simulink model "pfb_fir_generic_test_sim3"  (R2012b)
settings: Solver=VariableStepDiscrete  StartTime=0.0  StopTime=10.0  RelTol=1e-3
model workspace (MAT data in the model file):
  synci = [0 1 2 3 4 5 6 7 8 9 10 11 ... (589826 elements, 294913x2)]
  din0 = [0 1 2 3 4 5 6 7 8 9 10 11 ... (73730 elements, 36865x2)]
  din1 = [0 1 2 3 4 5 6 7 8 9 10 11 ... (73730 elements, 36865x2)]
  din2 = [0 1 2 3 4 5 6 7 8 9 10 11 ... (73730 elements, 36865x2)]
  din3 = [0 1 2 3 4 5 6 7 8 9 10 11 ... (73730 elements, 36865x2)]
  din4 = [0 1 2 3 4 5 6 7 8 9 10 11 ... (73730 elements, 36865x2)]
  din5 = [0 1 2 3 4 5 6 7 8 9 10 11 ... (73730 elements, 36865x2)]
  din6 = [0 1 2 3 4 5 6 7 8 9 10 11 ... (73730 elements, 36865x2)]
  din7 = [0 1 2 3 4 5 6 7 8 9 10 11 ... (73730 elements, 36865x2)]
libraries: xbsIndex_r4 x5585, casper_library_delays x1
(part 13 of 25)

== system pfb_fir_generic_test_sim3/pfb_fir_generic/pfb_fir_taps/delay_bram ==
  addr : Inport
  din : Inport  Port=2
  we : Inport  Port=3
  en : Inport  Port=4
  bram{0..26} (27 alike) : xbsIndex_r4/Single Port RAM  depth=1024  initVector=getfield(get_param(gcb, 'UserData'), 'initVector')  distributed_mem=Block RAM  write_mode=Read Before Write  rst=off  init_reg=0  en=on  latency=7  dbl_ovrd=off  optimize=Speed  block_type=spram
  ddin : xbsIndex_r4/Delay  rst=off  infoeditControl=Selection of Reset will increase slice count due to use of real FFs and instead of SRLs  en=off  latency=0  dbl_ovrd=off  reg_retiming=on  block_type=delay
  debus_addr : Subsystem  AncestorBlock=casper_library_flow_control/bus_expand  mask(bus_expand){mode=divisions of equal size, outputNum=27, outputWidth=[10 10 10 10 10 10 10 10 10 10 10 10 10 10 10 10 10 10 10 10 10 10 10 10 10 10 10], outputBinaryPt=[0 0 0 0 0 0 0 0 0 0 0 0 0 0 0 0 0 0 0 0 0 0 0 0 0 0 0], outputArithmeticType=[0 0 0 0 0 0 0 0 0 0 0 0 0 0 0 0 0 0 0 0 0 0 0 0 0 0 0], show_format=on, outputToWorkspace=off, variablePrefix=, outputToModelAsWell=on}
      mask prompts: outputNum "Number of outputs:"; outputWidth "Output width:"; outputBinaryPt "Output binary point position:"; outputArithmeticType "Output arithmetic type (ufix=0, fix=1, bool=2):"; show_format "Print format string?"; outputToWorkspace "Output to workspace?"; variablePrefix "Variable name prefix:"; outputToModelAsWell "Output to model as well?"
      mask help:
      | Expands a 'bus' made using a bus_create or Xilinx
      | concat block.
      | The input will be divided into the specified number
      | of outputs with the specified arithmetic types.
      | Divisions are made from most significant bit.
      mask init: same as pfb_fir_generic_test_sim3/pfb_fir_generic/bus_expand
      settings: AttributesFormatString=27 outputs: uf10.0,uf10.0,uf10.0,uf10.0,uf10.0,uf10.0,uf10.0,uf10.0,uf10.0,uf10.0,uf10.0,uf10.0,uf10.0,uf10.0,uf10.0,uf10.0,uf10.0,uf10.0,uf10.0,uf10.0,uf10.0,uf10.0,uf10.0,uf10.0,uf10.0,uf10.0,uf10.0,
      mask TypeOptions mode: divisions of equal size | divisions of arbitrary size
      mask Callback mode: bus_expand_callback();
      mask Callback outputWidth: bus_expand_callback();
      mask Callback outputToWorkspace: bus_expand_callback();
  debus_din : Subsystem  AncestorBlock=casper_library_flow_control/bus_expand  mask(bus_expand){mode=divisions of arbitrary size, outputNum=1, outputWidth=[12 18 18 18 18 18 18 18 18 18 18 18 18 18 18 18 18 18 18 18 18 18 18 18 18 18 18], outputBinaryPt=[0 0 0 0 0 0 0 0 0 0 0 0 0 0 0 0 0 0 0 0 0 0 0 0 0 0 0], outputArithmeticType=[0 0 0 0 0 0 0 0 0 0 0 0 0 0 0 0 0 0 0 0 0 0 0 0 0 0 0], show_format=on, outputToWorkspace=off, variablePrefix=, outputToModelAsWell=on}
      mask prompts: outputNum "Number of outputs:"; outputWidth "Output width [msb ... lsb]:"; outputBinaryPt "Output binary point position [msb ... lsb]:"; outputArithmeticType "Output arithmetic type (ufix=0, fix=1, bool=2) [msb ... lsb]:"; show_format "Print format string?"; outputToWorkspace "Output to workspace?"; variablePrefix "Variable name prefix:"; outputToModelAsWell "Output to model as well?"
      mask help:
      | Expands a 'bus' made using a bus_create or Xilinx
      | concat block.
      | The input will be divided into the specified number
      | of outputs with the specified arithmetic types.
      | Divisions are made from most significant bit.
      mask init: same as pfb_fir_generic_test_sim3/pfb_fir_generic/bus_expand
      settings: AttributesFormatString=27 outputs: uf12.0,uf18.0,uf18.0,uf18.0,uf18.0,uf18.0,uf18.0,uf18.0,uf18.0,uf18.0,uf18.0,uf18.0,uf18.0,uf18.0,uf18.0,uf18.0,uf18.0,uf18.0,uf18.0,uf18.0,uf18.0,uf18.0,uf18.0,uf18.0,uf18.0,uf18.0,uf18.0,
      mask TypeOptions mode: divisions of equal size | divisions of arbitrary size
      mask Callback mode: bus_expand_callback();
      mask Callback outputWidth: bus_expand_callback();
      mask Callback outputToWorkspace: bus_expand_callback();
  debus_en : Subsystem  AncestorBlock=casper_library_flow_control/bus_expand  mask(bus_expand){mode=divisions of equal size, outputNum=27, outputWidth=[1 1 1 1 1 1 1 1 1 1 1 1 1 1 1 1 1 1 1 1 1 1 1 1 1 1 1], outputBinaryPt=[0 0 0 0 0 0 0 0 0 0 0 0 0 0 0 0 0 0 0 0 0 0 0 0 0 0 0], outputArithmeticType=[2 2 2 2 2 2 2 2 2 2 2 2 2 2 2 2 2 2 2 2 2 2 2 2 2 2 2], show_format=on, outputToWorkspace=off, variablePrefix=, outputToModelAsWell=on}
      mask prompts: outputNum "Number of outputs:"; outputWidth "Output width:"; outputBinaryPt "Output binary point position:"; outputArithmeticType "Output arithmetic type (ufix=0, fix=1, bool=2):"; show_format "Print format string?"; outputToWorkspace "Output to workspace?"; variablePrefix "Variable name prefix:"; outputToModelAsWell "Output to model as well?"
      mask help:
      | Expands a 'bus' made using a bus_create or Xilinx
      | concat block.
      | The input will be divided into the specified number
      | of outputs with the specified arithmetic types.
      | Divisions are made from most significant bit.
      mask init: same as pfb_fir_generic_test_sim3/pfb_fir_generic/bus_expand
      settings: AttributesFormatString=27 outputs: b,b,b,b,b,b,b,b,b,b,b,b,b,b,b,b,b,b,b,b,b,b,b,b,b,b,b,
      mask TypeOptions mode: divisions of equal size | divisions of arbitrary size
      mask Callback mode: bus_expand_callback();
      mask Callback outputWidth: bus_expand_callback();
      mask Callback outputToWorkspace: bus_expand_callback();
  debus_we : Subsystem  AncestorBlock=casper_library_flow_control/bus_expand  mask(bus_expand){mode=divisions of equal size, outputNum=27, outputWidth=[1 1 1 1 1 1 1 1 1 1 1 1 1 1 1 1 1 1 1 1 1 1 1 1 1 1 1], outputBinaryPt=[0 0 0 0 0 0 0 0 0 0 0 0 0 0 0 0 0 0 0 0 0 0 0 0 0 0 0], outputArithmeticType=[2 2 2 2 2 2 2 2 2 2 2 2 2 2 2 2 2 2 2 2 2 2 2 2 2 2 2], show_format=on, outputToWorkspace=off, variablePrefix=, outputToModelAsWell=on}
      mask prompts: outputNum "Number of outputs:"; outputWidth "Output width:"; outputBinaryPt "Output binary point position:"; outputArithmeticType "Output arithmetic type (ufix=0, fix=1, bool=2):"; show_format "Print format string?"; outputToWorkspace "Output to workspace?"; variablePrefix "Variable name prefix:"; outputToModelAsWell "Output to model as well?"
      mask help:
      | Expands a 'bus' made using a bus_create or Xilinx
      | concat block.
      | The input will be divided into the specified number
      | of outputs with the specified arithmetic types.
      | Divisions are made from most significant bit.
      mask init: same as pfb_fir_generic_test_sim3/pfb_fir_generic/bus_expand
      settings: AttributesFormatString=27 outputs: b,b,b,b,b,b,b,b,b,b,b,b,b,b,b,b,b,b,b,b,b,b,b,b,b,b,b,
      mask TypeOptions mode: divisions of equal size | divisions of arbitrary size
      mask Callback mode: bus_expand_callback();
      mask Callback outputWidth: bus_expand_callback();
      mask Callback outputToWorkspace: bus_expand_callback();
  den : xbsIndex_r4/Delay  rst=off  infoeditControl=Selection of Reset will increase slice count due to use of real FFs and instead of SRLs  en=off  latency=7  dbl_ovrd=off  reg_retiming=on  block_type=delay
  din_bussify : Subsystem  AncestorBlock=casper_library_flow_control/bus_create  mask(bus_create){inputNum=27}
      mask prompts: inputNum "Number of inputs:"
      mask init:
      | bus_create_init(gcb,...
      |     'inputNum', inputNum);
  rep_addr : Subsystem  AncestorBlock=casper_library_bus/bus_replicate  mask(bus_replicate){replication=27, latency=9, misc=off, implementation=core}
      mask prompts: replication "replication factor"; misc "misc support"; implementation "delay implementation"
      mask help: Output bus formed by replicating input bus a number of times
      mask init:
      | bus_replicate_init(gcb, ...
      |     'replication', replication, ...
      |     'latency', latency, ...
      |     'implementation', implementation, ...
      |     'misc', misc);
      mask TypeOptions implementation: core | behavioral
  rep_en : Subsystem  AncestorBlock=casper_library_bus/bus_replicate  mask(bus_replicate){replication=27, latency=9, misc=off, implementation=core}
      mask prompts: replication "replication factor"; misc "misc support"; implementation "delay implementation"
      mask help: Output bus formed by replicating input bus a number of times
      mask init:
      | bus_replicate_init(gcb, ...
      |     'replication', replication, ...
      |     'latency', latency, ...
      |     'implementation', implementation, ...
      |     'misc', misc);
      mask TypeOptions implementation: core | behavioral
  rep_we : Subsystem  AncestorBlock=casper_library_bus/bus_replicate  mask(bus_replicate){replication=27, latency=0, misc=off, implementation=behavioral}
      mask prompts: replication "replication factor"; misc "misc support"; implementation "delay implementation"
      mask help: Output bus formed by replicating input bus a number of times
      mask init:
      | bus_replicate_init(gcb, ...
      |     'replication', replication, ...
      |     'latency', latency, ...
      |     'implementation', implementation, ...
      |     'misc', misc);
      mask TypeOptions implementation: core | behavioral
  dout : Outport
  dvalid : Outport  Port=2
  wires:
  addr/1 -> rep_addr/1(in)
  din/1 -> ddin/1
  we/1 -> rep_we/1(in)
  en/1 -> rep_en/1(in)
  rep_addr/1(out) -> debus_addr/1(bus_in)
  ddin/1 -> debus_din/1(bus_in)
  rep_we/1(out) -> debus_we/1(bus_in)
  rep_en/1(out) -> debus_en/1(bus_in)
  debus_addr/1(msb_out27) -> bram0/1
  debus_din/1(msb_out27) -> bram0/2
  debus_we/1(msb_out27) -> bram0/3
  debus_en/1(msb_out27) -> bram0/4
  debus_addr/2(out26) -> bram1/1
  debus_din/2(out26) -> bram1/2
  debus_we/2(out26) -> bram1/3
  debus_en/2(out26) -> bram1/4
  debus_addr/3(out25) -> bram2/1
  debus_din/3(out25) -> bram2/2
  debus_we/3(out25) -> bram2/3
  debus_en/3(out25) -> bram2/4
  debus_addr/4(out24) -> bram3/1
  debus_din/4(out24) -> bram3/2
  debus_we/4(out24) -> bram3/3
  debus_en/4(out24) -> bram3/4
  debus_addr/5(out23) -> bram4/1
  debus_din/5(out23) -> bram4/2
  debus_we/5(out23) -> bram4/3
  debus_en/5(out23) -> bram4/4
  debus_addr/6(out22) -> bram5/1
  debus_din/6(out22) -> bram5/2
  debus_we/6(out22) -> bram5/3
  debus_en/6(out22) -> bram5/4
  debus_addr/7(out21) -> bram6/1
  debus_din/7(out21) -> bram6/2
  debus_we/7(out21) -> bram6/3
  debus_en/7(out21) -> bram6/4
  debus_addr/8(out20) -> bram7/1
  debus_din/8(out20) -> bram7/2
  debus_we/8(out20) -> bram7/3
  debus_en/8(out20) -> bram7/4
  debus_addr/9(out19) -> bram8/1
  debus_din/9(out19) -> bram8/2
  debus_we/9(out19) -> bram8/3
  debus_en/9(out19) -> bram8/4
  debus_addr/10(out18) -> bram9/1
  debus_din/10(out18) -> bram9/2
  debus_we/10(out18) -> bram9/3
  debus_en/10(out18) -> bram9/4
  debus_addr/11(out17) -> bram10/1
  debus_din/11(out17) -> bram10/2
  debus_we/11(out17) -> bram10/3
  debus_en/11(out17) -> bram10/4
  debus_addr/12(out16) -> bram11/1
  debus_din/12(out16) -> bram11/2
  debus_we/12(out16) -> bram11/3
  debus_en/12(out16) -> bram11/4
  debus_addr/13(out15) -> bram12/1
  debus_din/13(out15) -> bram12/2
  debus_we/13(out15) -> bram12/3
  debus_en/13(out15) -> bram12/4
  debus_addr/14(out14) -> bram13/1
  debus_din/14(out14) -> bram13/2
  debus_we/14(out14) -> bram13/3
  debus_en/14(out14) -> bram13/4
  debus_addr/15(out13) -> bram14/1
  debus_din/15(out13) -> bram14/2
  debus_we/15(out13) -> bram14/3
  debus_en/15(out13) -> bram14/4
  debus_addr/16(out12) -> bram15/1
  debus_din/16(out12) -> bram15/2
  debus_we/16(out12) -> bram15/3
  debus_en/16(out12) -> bram15/4
  debus_addr/17(out11) -> bram16/1
  debus_din/17(out11) -> bram16/2
  debus_we/17(out11) -> bram16/3
  debus_en/17(out11) -> bram16/4
  debus_addr/18(out10) -> bram17/1
  debus_din/18(out10) -> bram17/2
  debus_we/18(out10) -> bram17/3
  debus_en/18(out10) -> bram17/4
  debus_addr/19(out9) -> bram18/1
  debus_din/19(out9) -> bram18/2
  debus_we/19(out9) -> bram18/3
  debus_en/19(out9) -> bram18/4
  debus_addr/20(out8) -> bram19/1
  debus_din/20(out8) -> bram19/2
  debus_we/20(out8) -> bram19/3
  debus_en/20(out8) -> bram19/4
  debus_addr/21(out7) -> bram20/1
  debus_din/21(out7) -> bram20/2
  debus_we/21(out7) -> bram20/3
  debus_en/21(out7) -> bram20/4
  debus_addr/22(out6) -> bram21/1
  debus_din/22(out6) -> bram21/2
  debus_we/22(out6) -> bram21/3
  debus_en/22(out6) -> bram21/4
  debus_addr/23(out5) -> bram22/1
  debus_din/23(out5) -> bram22/2
  debus_we/23(out5) -> bram22/3
  debus_en/23(out5) -> bram22/4
  debus_addr/24(out4) -> bram23/1
  debus_din/24(out4) -> bram23/2
  debus_we/24(out4) -> bram23/3
  debus_en/24(out4) -> bram23/4
  debus_addr/25(out3) -> bram24/1
  debus_din/25(out3) -> bram24/2
  debus_we/25(out3) -> bram24/3
  debus_en/25(out3) -> bram24/4
  debus_addr/26(out2) -> bram25/1
  debus_din/26(out2) -> bram25/2
  debus_we/26(out2) -> bram25/3
  debus_en/26(out2) -> bram25/4
  debus_addr/27(lsb_out1) -> bram26/1
  debus_din/27(lsb_out1) -> bram26/2
  debus_we/27(lsb_out1) -> bram26/3
  debus_en/27(lsb_out1) -> bram26/4, den/1
  bram0/1 -> din_bussify/1(in1)
  bram1/1 -> din_bussify/2(in2)
  bram2/1 -> din_bussify/3(in3)
  bram3/1 -> din_bussify/4(in4)
  bram4/1 -> din_bussify/5(in5)
  bram5/1 -> din_bussify/6(in6)
  bram6/1 -> din_bussify/7(in7)
  bram7/1 -> din_bussify/8(in8)
  bram8/1 -> din_bussify/9(in9)
  bram9/1 -> din_bussify/10(in10)
  bram10/1 -> din_bussify/11(in11)
  bram11/1 -> din_bussify/12(in12)
  bram12/1 -> din_bussify/13(in13)
  bram13/1 -> din_bussify/14(in14)
  bram14/1 -> din_bussify/15(in15)
  bram15/1 -> din_bussify/16(in16)
  bram16/1 -> din_bussify/17(in17)
  bram17/1 -> din_bussify/18(in18)
  bram18/1 -> din_bussify/19(in19)
  bram19/1 -> din_bussify/20(in20)
  bram20/1 -> din_bussify/21(in21)
  bram21/1 -> din_bussify/22(in22)
  bram22/1 -> din_bussify/23(in23)
  bram23/1 -> din_bussify/24(in24)
  bram24/1 -> din_bussify/25(in25)
  bram25/1 -> din_bussify/26(in26)
  bram26/1 -> din_bussify/27(in27)
  din_bussify/1(bus_out) -> dout/1
  den/1 -> dvalid/1

== system pfb_fir_generic_test_sim3/pfb_fir_generic/pfb_fir_taps/en_expand ==
  bus_in : Inport
  slice1 : xbsIndex_r4/Slice  nbits=1  boolean_output=on  mode=Upper Bit Location + Width  bit1=-1  base1=MSB of Input  bit0=0  base0=LSB of Input  dbl_ovrd=off  block_type=slice
  slice2 : xbsIndex_r4/Slice  nbits=1  boolean_output=on  mode=Upper Bit Location + Width  bit1=0  base1=MSB of Input  bit0=0  base0=LSB of Input  dbl_ovrd=off  block_type=slice
  msb_out2 : Outport
  lsb_out1 : Outport  Port=2
  wires:
  bus_in/1 -> slice2/1, slice1/1
  slice2/1 -> msb_out2/1
  slice1/1 -> lsb_out1/1

== system pfb_fir_generic_test_sim3/pfb_fir_generic/pfb_fir_taps/en_replicate0 ==
  in : Inport
  bussify : Subsystem  AncestorBlock=casper_library_flow_control/bus_create  mask(bus_create){inputNum=48}
      mask prompts: inputNum "Number of inputs:"
      mask init:
      | bus_create_init(gcb,...
      |     'inputNum', inputNum);
  din0_0 : xbsIndex_r4/Delay  rst=off  infoeditControl=Selection of Reset will increase slice count due to use of real FFs and instead of SRLs  en=off  latency=1  dbl_ovrd=off  reg_retiming=off  block_type=delay
  din1_0 : xbsIndex_r4/Delay  rst=off  infoeditControl=Selection of Reset will increase slice count due to use of real FFs and instead of SRLs  en=off  latency=1  dbl_ovrd=off  reg_retiming=off  block_type=delay
  din1_1 : xbsIndex_r4/Delay  rst=off  infoeditControl=Selection of Reset will increase slice count due to use of real FFs and instead of SRLs  en=off  latency=1  dbl_ovrd=off  reg_retiming=off  block_type=delay
  din2_{0..3} (4 alike) : xbsIndex_r4/Delay  rst=off  infoeditControl=Selection of Reset will increase slice count due to use of real FFs and instead of SRLs  en=off  latency=1  dbl_ovrd=off  reg_retiming=off  block_type=delay
  din3_{0..7} (8 alike) : xbsIndex_r4/Delay  rst=off  infoeditControl=Selection of Reset will increase slice count due to use of real FFs and instead of SRLs  en=off  latency=1  dbl_ovrd=off  reg_retiming=off  block_type=delay
  din4_{0..15} (16 alike) : xbsIndex_r4/Delay  rst=off  infoeditControl=Selection of Reset will increase slice count due to use of real FFs and instead of SRLs  en=off  latency=1  dbl_ovrd=off  reg_retiming=off  block_type=delay
  din5_{0..31} (32 alike) : xbsIndex_r4/Delay  rst=off  infoeditControl=Selection of Reset will increase slice count due to use of real FFs and instead of SRLs  en=off  latency=1  dbl_ovrd=off  reg_retiming=off  block_type=delay
  din6_{0..47} (48 alike) : xbsIndex_r4/Delay  rst=off  infoeditControl=Selection of Reset will increase slice count due to use of real FFs and instead of SRLs  en=off  latency=1  dbl_ovrd=off  reg_retiming=on  block_type=delay
  din7_{0..47} (48 alike) : xbsIndex_r4/Delay  rst=off  infoeditControl=Selection of Reset will increase slice count due to use of real FFs and instead of SRLs  en=off  latency=1  dbl_ovrd=off  reg_retiming=on  block_type=delay
  din8_{0..47} (48 alike) : xbsIndex_r4/Delay  rst=off  infoeditControl=Selection of Reset will increase slice count due to use of real FFs and instead of SRLs  en=off  latency=1  dbl_ovrd=off  reg_retiming=off  block_type=delay
  out : Outport
  wires:
  in/1 -> din0_0/1
  din0_0/1 -> din1_0/1, din1_1/1
  din1_0/1 -> din2_0/1, din2_2/1
  din1_1/1 -> din2_1/1, din2_3/1
  din2_0/1 -> din3_0/1, din3_4/1
  din2_1/1 -> din3_1/1, din3_5/1
  din2_2/1 -> din3_2/1, din3_6/1
  din2_3/1 -> din3_3/1, din3_7/1
  din3_0/1 -> din4_0/1, din4_8/1
  din3_1/1 -> din4_1/1, din4_9/1
  din3_2/1 -> din4_2/1, din4_10/1
  din3_3/1 -> din4_3/1, din4_11/1
  din3_4/1 -> din4_4/1, din4_12/1
  din3_5/1 -> din4_5/1, din4_13/1
  din3_6/1 -> din4_6/1, din4_14/1
  din3_7/1 -> din4_7/1, din4_15/1
  din4_0/1 -> din5_0/1, din5_16/1
  din4_1/1 -> din5_1/1, din5_17/1
  din4_2/1 -> din5_2/1, din5_18/1
  din4_3/1 -> din5_3/1, din5_19/1
  din4_4/1 -> din5_4/1, din5_20/1
  din4_5/1 -> din5_5/1, din5_21/1
  din4_6/1 -> din5_6/1, din5_22/1
  din4_7/1 -> din5_7/1, din5_23/1
  din4_8/1 -> din5_8/1, din5_24/1
  din4_9/1 -> din5_9/1, din5_25/1
  din4_10/1 -> din5_10/1, din5_26/1
  din4_11/1 -> din5_11/1, din5_27/1
  din4_12/1 -> din5_12/1, din5_28/1
  din4_13/1 -> din5_13/1, din5_29/1
  din4_14/1 -> din5_14/1, din5_30/1
  din4_15/1 -> din5_15/1, din5_31/1
  din5_0/1 -> din6_0/1, din6_32/1
  din5_1/1 -> din6_1/1, din6_33/1
  din5_2/1 -> din6_2/1, din6_34/1
  din5_3/1 -> din6_3/1, din6_35/1
  din5_4/1 -> din6_4/1, din6_36/1
  din5_5/1 -> din6_5/1, din6_37/1
  din5_6/1 -> din6_6/1, din6_38/1
  din5_7/1 -> din6_7/1, din6_39/1
  din5_8/1 -> din6_8/1, din6_40/1
  din5_9/1 -> din6_9/1, din6_41/1
  din5_10/1 -> din6_10/1, din6_42/1
  din5_11/1 -> din6_11/1, din6_43/1
  din5_12/1 -> din6_12/1, din6_44/1
  din5_13/1 -> din6_13/1, din6_45/1
  din5_14/1 -> din6_14/1, din6_46/1
  din5_15/1 -> din6_15/1, din6_47/1
  din5_16/1 -> din6_16/1
  din5_17/1 -> din6_17/1
  din5_18/1 -> din6_18/1
  din5_19/1 -> din6_19/1
  din5_20/1 -> din6_20/1
  din5_21/1 -> din6_21/1
  din5_22/1 -> din6_22/1
  din5_23/1 -> din6_23/1
  din5_24/1 -> din6_24/1
  din5_25/1 -> din6_25/1
  din5_26/1 -> din6_26/1
  din5_27/1 -> din6_27/1
  din5_28/1 -> din6_28/1
  din5_29/1 -> din6_29/1
  din5_30/1 -> din6_30/1
  din5_31/1 -> din6_31/1
  din6_0/1 -> din7_0/1
  din6_1/1 -> din7_1/1
  din6_2/1 -> din7_2/1
  din6_3/1 -> din7_3/1
  din6_4/1 -> din7_4/1
  din6_5/1 -> din7_5/1
  din6_6/1 -> din7_6/1
  din6_7/1 -> din7_7/1
  din6_8/1 -> din7_8/1
  din6_9/1 -> din7_9/1
  din6_10/1 -> din7_10/1
  din6_11/1 -> din7_11/1
  din6_12/1 -> din7_12/1
  din6_13/1 -> din7_13/1
  din6_14/1 -> din7_14/1
  din6_15/1 -> din7_15/1
  din6_16/1 -> din7_16/1
  din6_17/1 -> din7_17/1
  din6_18/1 -> din7_18/1
  din6_19/1 -> din7_19/1
  din6_20/1 -> din7_20/1
  din6_21/1 -> din7_21/1
  din6_22/1 -> din7_22/1
  din6_23/1 -> din7_23/1
  din6_24/1 -> din7_24/1
  din6_25/1 -> din7_25/1
  din6_26/1 -> din7_26/1
  din6_27/1 -> din7_27/1
  din6_28/1 -> din7_28/1
  din6_29/1 -> din7_29/1
  din6_30/1 -> din7_30/1
  din6_31/1 -> din7_31/1
  din6_32/1 -> din7_32/1
  din6_33/1 -> din7_33/1
  din6_34/1 -> din7_34/1
  din6_35/1 -> din7_35/1
  din6_36/1 -> din7_36/1
  din6_37/1 -> din7_37/1
  din6_38/1 -> din7_38/1
  din6_39/1 -> din7_39/1
  din6_40/1 -> din7_40/1
  din6_41/1 -> din7_41/1
  din6_42/1 -> din7_42/1
  din6_43/1 -> din7_43/1
  din6_44/1 -> din7_44/1
  din6_45/1 -> din7_45/1
  din6_46/1 -> din7_46/1
  din6_47/1 -> din7_47/1
  din7_0/1 -> din8_0/1
  din7_1/1 -> din8_1/1
  din7_2/1 -> din8_2/1
  din7_3/1 -> din8_3/1
  din7_4/1 -> din8_4/1
  din7_5/1 -> din8_5/1
  din7_6/1 -> din8_6/1
  din7_7/1 -> din8_7/1
  din7_8/1 -> din8_8/1
  din7_9/1 -> din8_9/1
  din7_10/1 -> din8_10/1
  din7_11/1 -> din8_11/1
  din7_12/1 -> din8_12/1
  din7_13/1 -> din8_13/1
  din7_14/1 -> din8_14/1
  din7_15/1 -> din8_15/1
  din7_16/1 -> din8_16/1
  din7_17/1 -> din8_17/1
  din7_18/1 -> din8_18/1
  din7_19/1 -> din8_19/1
  din7_20/1 -> din8_20/1
  din7_21/1 -> din8_21/1
  din7_22/1 -> din8_22/1
  din7_23/1 -> din8_23/1
  din7_24/1 -> din8_24/1
  din7_25/1 -> din8_25/1
  din7_26/1 -> din8_26/1
  din7_27/1 -> din8_27/1
  din7_28/1 -> din8_28/1
  din7_29/1 -> din8_29/1
  din7_30/1 -> din8_30/1
  din7_31/1 -> din8_31/1
  din7_32/1 -> din8_32/1
  din7_33/1 -> din8_33/1
  din7_34/1 -> din8_34/1
  din7_35/1 -> din8_35/1
  din7_36/1 -> din8_36/1
  din7_37/1 -> din8_37/1
  din7_38/1 -> din8_38/1
  din7_39/1 -> din8_39/1
  din7_40/1 -> din8_40/1
  din7_41/1 -> din8_41/1
  din7_42/1 -> din8_42/1
  din7_43/1 -> din8_43/1
  din7_44/1 -> din8_44/1
  din7_45/1 -> din8_45/1
  din7_46/1 -> din8_46/1
  din7_47/1 -> din8_47/1
  din8_0/1 -> bussify/1(in1)
  din8_1/1 -> bussify/2(in2)
  din8_2/1 -> bussify/3(in3)
  din8_3/1 -> bussify/4(in4)
  din8_4/1 -> bussify/5(in5)
  din8_5/1 -> bussify/6(in6)
  din8_6/1 -> bussify/7(in7)
  din8_7/1 -> bussify/8(in8)
  din8_8/1 -> bussify/9(in9)
  din8_9/1 -> bussify/10(in10)
  din8_10/1 -> bussify/11(in11)
  din8_11/1 -> bussify/12(in12)
  din8_12/1 -> bussify/13(in13)
  din8_13/1 -> bussify/14(in14)
  din8_14/1 -> bussify/15(in15)
  din8_15/1 -> bussify/16(in16)
  din8_16/1 -> bussify/17(in17)
  din8_17/1 -> bussify/18(in18)
  din8_18/1 -> bussify/19(in19)
  din8_19/1 -> bussify/20(in20)
  din8_20/1 -> bussify/21(in21)
  din8_21/1 -> bussify/22(in22)
  din8_22/1 -> bussify/23(in23)
  din8_23/1 -> bussify/24(in24)
  din8_24/1 -> bussify/25(in25)
  din8_25/1 -> bussify/26(in26)
  din8_26/1 -> bussify/27(in27)
  din8_27/1 -> bussify/28(in28)
  din8_28/1 -> bussify/29(in29)
  din8_29/1 -> bussify/30(in30)
  din8_30/1 -> bussify/31(in31)
  din8_31/1 -> bussify/32(in32)
  din8_32/1 -> bussify/33(in33)
  din8_33/1 -> bussify/34(in34)
  din8_34/1 -> bussify/35(in35)
  din8_35/1 -> bussify/36(in36)
  din8_36/1 -> bussify/37(in37)
  din8_37/1 -> bussify/38(in38)
  din8_38/1 -> bussify/39(in39)
  din8_39/1 -> bussify/40(in40)
  din8_40/1 -> bussify/41(in41)
  din8_41/1 -> bussify/42(in42)
  din8_42/1 -> bussify/43(in43)
  din8_43/1 -> bussify/44(in44)
  din8_44/1 -> bussify/45(in45)
  din8_45/1 -> bussify/46(in46)
  din8_46/1 -> bussify/47(in47)
  din8_47/1 -> bussify/48(in48)
  bussify/1(bus_out) -> out/1

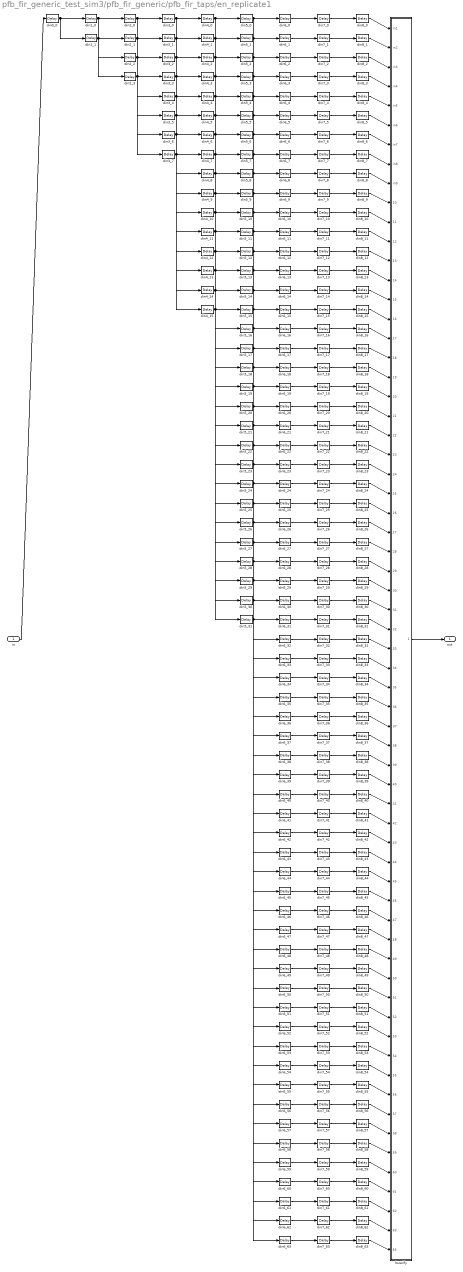
== system pfb_fir_generic_test_sim3/pfb_fir_generic/pfb_fir_taps/en_replicate1 ==
  in : Inport
  bussify : Subsystem  AncestorBlock=casper_library_flow_control/bus_create  mask(bus_create){inputNum=64}
      mask prompts: inputNum "Number of inputs:"
      mask init:
      | bus_create_init(gcb,...
      |     'inputNum', inputNum);
  din0_0 : xbsIndex_r4/Delay  rst=off  infoeditControl=Selection of Reset will increase slice count due to use of real FFs and instead of SRLs  en=off  latency=1  dbl_ovrd=off  reg_retiming=off  block_type=delay
  din1_0 : xbsIndex_r4/Delay  rst=off  infoeditControl=Selection of Reset will increase slice count due to use of real FFs and instead of SRLs  en=off  latency=1  dbl_ovrd=off  reg_retiming=off  block_type=delay
  din1_1 : xbsIndex_r4/Delay  rst=off  infoeditControl=Selection of Reset will increase slice count due to use of real FFs and instead of SRLs  en=off  latency=1  dbl_ovrd=off  reg_retiming=off  block_type=delay
  din2_{0..3} (4 alike) : xbsIndex_r4/Delay  rst=off  infoeditControl=Selection of Reset will increase slice count due to use of real FFs and instead of SRLs  en=off  latency=1  dbl_ovrd=off  reg_retiming=off  block_type=delay
  din3_{0..7} (8 alike) : xbsIndex_r4/Delay  rst=off  infoeditControl=Selection of Reset will increase slice count due to use of real FFs and instead of SRLs  en=off  latency=1  dbl_ovrd=off  reg_retiming=off  block_type=delay
  din4_{0..15} (16 alike) : xbsIndex_r4/Delay  rst=off  infoeditControl=Selection of Reset will increase slice count due to use of real FFs and instead of SRLs  en=off  latency=1  dbl_ovrd=off  reg_retiming=off  block_type=delay
  din5_{0..31} (32 alike) : xbsIndex_r4/Delay  rst=off  infoeditControl=Selection of Reset will increase slice count due to use of real FFs and instead of SRLs  en=off  latency=1  dbl_ovrd=off  reg_retiming=off  block_type=delay
  din6_{0..63} (64 alike) : xbsIndex_r4/Delay  rst=off  infoeditControl=Selection of Reset will increase slice count due to use of real FFs and instead of SRLs  en=off  latency=1  dbl_ovrd=off  reg_retiming=on  block_type=delay
  din7_{0..63} (64 alike) : xbsIndex_r4/Delay  rst=off  infoeditControl=Selection of Reset will increase slice count due to use of real FFs and instead of SRLs  en=off  latency=1  dbl_ovrd=off  reg_retiming=on  block_type=delay
  din8_{0..63} (64 alike) : xbsIndex_r4/Delay  rst=off  infoeditControl=Selection of Reset will increase slice count due to use of real FFs and instead of SRLs  en=off  latency=1  dbl_ovrd=off  reg_retiming=off  block_type=delay
  out : Outport
  wires:
  in/1 -> din0_0/1
  din0_0/1 -> din1_0/1, din1_1/1
  din1_0/1 -> din2_0/1, din2_2/1
  din1_1/1 -> din2_1/1, din2_3/1
  din2_0/1 -> din3_0/1, din3_4/1
  din2_1/1 -> din3_1/1, din3_5/1
  din2_2/1 -> din3_2/1, din3_6/1
  din2_3/1 -> din3_3/1, din3_7/1
  din3_0/1 -> din4_0/1, din4_8/1
  din3_1/1 -> din4_1/1, din4_9/1
  din3_2/1 -> din4_2/1, din4_10/1
  din3_3/1 -> din4_3/1, din4_11/1
  din3_4/1 -> din4_4/1, din4_12/1
  din3_5/1 -> din4_5/1, din4_13/1
  din3_6/1 -> din4_6/1, din4_14/1
  din3_7/1 -> din4_7/1, din4_15/1
  din4_0/1 -> din5_0/1, din5_16/1
  din4_1/1 -> din5_1/1, din5_17/1
  din4_2/1 -> din5_2/1, din5_18/1
  din4_3/1 -> din5_3/1, din5_19/1
  din4_4/1 -> din5_4/1, din5_20/1
  din4_5/1 -> din5_5/1, din5_21/1
  din4_6/1 -> din5_6/1, din5_22/1
  din4_7/1 -> din5_7/1, din5_23/1
  din4_8/1 -> din5_8/1, din5_24/1
  din4_9/1 -> din5_9/1, din5_25/1
  din4_10/1 -> din5_10/1, din5_26/1
  din4_11/1 -> din5_11/1, din5_27/1
  din4_12/1 -> din5_12/1, din5_28/1
  din4_13/1 -> din5_13/1, din5_29/1
  din4_14/1 -> din5_14/1, din5_30/1
  din4_15/1 -> din5_15/1, din5_31/1
  din5_0/1 -> din6_0/1, din6_32/1
  din5_1/1 -> din6_1/1, din6_33/1
  din5_2/1 -> din6_2/1, din6_34/1
  din5_3/1 -> din6_3/1, din6_35/1
  din5_4/1 -> din6_4/1, din6_36/1
  din5_5/1 -> din6_5/1, din6_37/1
  din5_6/1 -> din6_6/1, din6_38/1
  din5_7/1 -> din6_7/1, din6_39/1
  din5_8/1 -> din6_8/1, din6_40/1
  din5_9/1 -> din6_9/1, din6_41/1
  din5_10/1 -> din6_10/1, din6_42/1
  din5_11/1 -> din6_11/1, din6_43/1
  din5_12/1 -> din6_12/1, din6_44/1
  din5_13/1 -> din6_13/1, din6_45/1
  din5_14/1 -> din6_14/1, din6_46/1
  din5_15/1 -> din6_15/1, din6_47/1
  din5_16/1 -> din6_16/1, din6_48/1
  din5_17/1 -> din6_17/1, din6_49/1
  din5_18/1 -> din6_18/1, din6_50/1
  din5_19/1 -> din6_19/1, din6_51/1
  din5_20/1 -> din6_20/1, din6_52/1
  din5_21/1 -> din6_21/1, din6_53/1
  din5_22/1 -> din6_22/1, din6_54/1
  din5_23/1 -> din6_23/1, din6_55/1
  din5_24/1 -> din6_24/1, din6_56/1
  din5_25/1 -> din6_25/1, din6_57/1
  din5_26/1 -> din6_26/1, din6_58/1
  din5_27/1 -> din6_27/1, din6_59/1
  din5_28/1 -> din6_28/1, din6_60/1
  din5_29/1 -> din6_29/1, din6_61/1
  din5_30/1 -> din6_30/1, din6_62/1
  din5_31/1 -> din6_31/1, din6_63/1
  din6_0/1 -> din7_0/1
  din6_1/1 -> din7_1/1
  din6_2/1 -> din7_2/1
  din6_3/1 -> din7_3/1
  din6_4/1 -> din7_4/1
  din6_5/1 -> din7_5/1
  din6_6/1 -> din7_6/1
  din6_7/1 -> din7_7/1
  din6_8/1 -> din7_8/1
  din6_9/1 -> din7_9/1
  din6_10/1 -> din7_10/1
  din6_11/1 -> din7_11/1
  din6_12/1 -> din7_12/1
  din6_13/1 -> din7_13/1
  din6_14/1 -> din7_14/1
  din6_15/1 -> din7_15/1
  din6_16/1 -> din7_16/1
  din6_17/1 -> din7_17/1
  din6_18/1 -> din7_18/1
  din6_19/1 -> din7_19/1
  din6_20/1 -> din7_20/1
  din6_21/1 -> din7_21/1
  din6_22/1 -> din7_22/1
  din6_23/1 -> din7_23/1
  din6_24/1 -> din7_24/1
  din6_25/1 -> din7_25/1
  din6_26/1 -> din7_26/1
  din6_27/1 -> din7_27/1
  din6_28/1 -> din7_28/1
  din6_29/1 -> din7_29/1
  din6_30/1 -> din7_30/1
  din6_31/1 -> din7_31/1
  din6_32/1 -> din7_32/1
  din6_33/1 -> din7_33/1
  din6_34/1 -> din7_34/1
  din6_35/1 -> din7_35/1
  din6_36/1 -> din7_36/1
  din6_37/1 -> din7_37/1
  din6_38/1 -> din7_38/1
  din6_39/1 -> din7_39/1
  din6_40/1 -> din7_40/1
  din6_41/1 -> din7_41/1
  din6_42/1 -> din7_42/1
  din6_43/1 -> din7_43/1
  din6_44/1 -> din7_44/1
  din6_45/1 -> din7_45/1
  din6_46/1 -> din7_46/1
  din6_47/1 -> din7_47/1
  din6_48/1 -> din7_48/1
  din6_49/1 -> din7_49/1
  din6_50/1 -> din7_50/1
  din6_51/1 -> din7_51/1
  din6_52/1 -> din7_52/1
  din6_53/1 -> din7_53/1
  din6_54/1 -> din7_54/1
  din6_55/1 -> din7_55/1
  din6_56/1 -> din7_56/1
  din6_57/1 -> din7_57/1
  din6_58/1 -> din7_58/1
  din6_59/1 -> din7_59/1
  din6_60/1 -> din7_60/1
  din6_61/1 -> din7_61/1
  din6_62/1 -> din7_62/1
  din6_63/1 -> din7_63/1
  din7_0/1 -> din8_0/1
  din7_1/1 -> din8_1/1
  din7_2/1 -> din8_2/1
  din7_3/1 -> din8_3/1
  din7_4/1 -> din8_4/1
  din7_5/1 -> din8_5/1
  din7_6/1 -> din8_6/1
  din7_7/1 -> din8_7/1
  din7_8/1 -> din8_8/1
  din7_9/1 -> din8_9/1
  din7_10/1 -> din8_10/1
  din7_11/1 -> din8_11/1
  din7_12/1 -> din8_12/1
  din7_13/1 -> din8_13/1
  din7_14/1 -> din8_14/1
  din7_15/1 -> din8_15/1
  din7_16/1 -> din8_16/1
  din7_17/1 -> din8_17/1
  din7_18/1 -> din8_18/1
  din7_19/1 -> din8_19/1
  din7_20/1 -> din8_20/1
  din7_21/1 -> din8_21/1
  din7_22/1 -> din8_22/1
  din7_23/1 -> din8_23/1
  din7_24/1 -> din8_24/1
  din7_25/1 -> din8_25/1
  din7_26/1 -> din8_26/1
  din7_27/1 -> din8_27/1
  din7_28/1 -> din8_28/1
  din7_29/1 -> din8_29/1
  din7_30/1 -> din8_30/1
  din7_31/1 -> din8_31/1
  din7_32/1 -> din8_32/1
  din7_33/1 -> din8_33/1
  din7_34/1 -> din8_34/1
  din7_35/1 -> din8_35/1
  din7_36/1 -> din8_36/1
  din7_37/1 -> din8_37/1
  din7_38/1 -> din8_38/1
  din7_39/1 -> din8_39/1
  din7_40/1 -> din8_40/1
  din7_41/1 -> din8_41/1
  din7_42/1 -> din8_42/1
  din7_43/1 -> din8_43/1
  din7_44/1 -> din8_44/1
  din7_45/1 -> din8_45/1
  din7_46/1 -> din8_46/1
  din7_47/1 -> din8_47/1
  din7_48/1 -> din8_48/1
  din7_49/1 -> din8_49/1
  din7_50/1 -> din8_50/1
  din7_51/1 -> din8_51/1
  din7_52/1 -> din8_52/1
  din7_53/1 -> din8_53/1
  din7_54/1 -> din8_54/1
  din7_55/1 -> din8_55/1
  din7_56/1 -> din8_56/1
  din7_57/1 -> din8_57/1
  din7_58/1 -> din8_58/1
  din7_59/1 -> din8_59/1
  din7_60/1 -> din8_60/1
  din7_61/1 -> din8_61/1
  din7_62/1 -> din8_62/1
  din7_63/1 -> din8_63/1
  din8_0/1 -> bussify/1(in1)
  din8_1/1 -> bussify/2(in2)
  din8_2/1 -> bussify/3(in3)
  din8_3/1 -> bussify/4(in4)
  din8_4/1 -> bussify/5(in5)
  din8_5/1 -> bussify/6(in6)
  din8_6/1 -> bussify/7(in7)
  din8_7/1 -> bussify/8(in8)
  din8_8/1 -> bussify/9(in9)
  din8_9/1 -> bussify/10(in10)
  din8_10/1 -> bussify/11(in11)
  din8_11/1 -> bussify/12(in12)
  din8_12/1 -> bussify/13(in13)
  din8_13/1 -> bussify/14(in14)
  din8_14/1 -> bussify/15(in15)
  din8_15/1 -> bussify/16(in16)
  din8_16/1 -> bussify/17(in17)
  din8_17/1 -> bussify/18(in18)
  din8_18/1 -> bussify/19(in19)
  din8_19/1 -> bussify/20(in20)
  din8_20/1 -> bussify/21(in21)
  din8_21/1 -> bussify/22(in22)
  din8_22/1 -> bussify/23(in23)
  din8_23/1 -> bussify/24(in24)
  din8_24/1 -> bussify/25(in25)
  din8_25/1 -> bussify/26(in26)
  din8_26/1 -> bussify/27(in27)
  din8_27/1 -> bussify/28(in28)
  din8_28/1 -> bussify/29(in29)
  din8_29/1 -> bussify/30(in30)
  din8_30/1 -> bussify/31(in31)
  din8_31/1 -> bussify/32(in32)
  din8_32/1 -> bussify/33(in33)
  din8_33/1 -> bussify/34(in34)
  din8_34/1 -> bussify/35(in35)
  din8_35/1 -> bussify/36(in36)
  din8_36/1 -> bussify/37(in37)
  din8_37/1 -> bussify/38(in38)
  din8_38/1 -> bussify/39(in39)
  din8_39/1 -> bussify/40(in40)
  din8_40/1 -> bussify/41(in41)
  din8_41/1 -> bussify/42(in42)
  din8_42/1 -> bussify/43(in43)
  din8_43/1 -> bussify/44(in44)
  din8_44/1 -> bussify/45(in45)
  din8_45/1 -> bussify/46(in46)
  din8_46/1 -> bussify/47(in47)
  din8_47/1 -> bussify/48(in48)
  din8_48/1 -> bussify/49(in49)
  din8_49/1 -> bussify/50(in50)
  din8_50/1 -> bussify/51(in51)
  din8_51/1 -> bussify/52(in52)
  din8_52/1 -> bussify/53(in53)
  din8_53/1 -> bussify/54(in54)
  din8_54/1 -> bussify/55(in55)
  din8_55/1 -> bussify/56(in56)
  din8_56/1 -> bussify/57(in57)
  din8_57/1 -> bussify/58(in58)
  din8_58/1 -> bussify/59(in59)
  din8_59/1 -> bussify/60(in60)
  din8_60/1 -> bussify/61(in61)
  din8_61/1 -> bussify/62(in62)
  din8_62/1 -> bussify/63(in63)
  din8_63/1 -> bussify/64(in64)
  bussify/1(bus_out) -> out/1

== system pfb_fir_generic_test_sim3/pfb_fir_generic/pfb_fir_taps/en_replicate2 ==
  in : Inport
  bussify : Subsystem  AncestorBlock=casper_library_flow_control/bus_create  mask(bus_create){inputNum=2}
      mask prompts: inputNum "Number of inputs:"
      mask init:
      | bus_create_init(gcb,...
      |     'inputNum', inputNum);
  din0_0 : xbsIndex_r4/Delay  rst=off  infoeditControl=Selection of Reset will increase slice count due to use of real FFs and instead of SRLs  en=off  latency=1  dbl_ovrd=off  reg_retiming=off  block_type=delay
  din1_0 : xbsIndex_r4/Delay  rst=off  infoeditControl=Selection of Reset will increase slice count due to use of real FFs and instead of SRLs  en=off  latency=1  dbl_ovrd=off  reg_retiming=on  block_type=delay
  din1_1 : xbsIndex_r4/Delay  rst=off  infoeditControl=Selection of Reset will increase slice count due to use of real FFs and instead of SRLs  en=off  latency=1  dbl_ovrd=off  reg_retiming=on  block_type=delay
  din2_0 : xbsIndex_r4/Delay  rst=off  infoeditControl=Selection of Reset will increase slice count due to use of real FFs and instead of SRLs  en=off  latency=1  dbl_ovrd=off  reg_retiming=on  block_type=delay
  din2_1 : xbsIndex_r4/Delay  rst=off  infoeditControl=Selection of Reset will increase slice count due to use of real FFs and instead of SRLs  en=off  latency=1  dbl_ovrd=off  reg_retiming=on  block_type=delay
  din3_0 : xbsIndex_r4/Delay  rst=off  infoeditControl=Selection of Reset will increase slice count due to use of real FFs and instead of SRLs  en=off  latency=1  dbl_ovrd=off  reg_retiming=on  block_type=delay
  din3_1 : xbsIndex_r4/Delay  rst=off  infoeditControl=Selection of Reset will increase slice count due to use of real FFs and instead of SRLs  en=off  latency=1  dbl_ovrd=off  reg_retiming=on  block_type=delay
  din4_0 : xbsIndex_r4/Delay  rst=off  infoeditControl=Selection of Reset will increase slice count due to use of real FFs and instead of SRLs  en=off  latency=1  dbl_ovrd=off  reg_retiming=on  block_type=delay
  din4_1 : xbsIndex_r4/Delay  rst=off  infoeditControl=Selection of Reset will increase slice count due to use of real FFs and instead of SRLs  en=off  latency=1  dbl_ovrd=off  reg_retiming=on  block_type=delay
  din5_0 : xbsIndex_r4/Delay  rst=off  infoeditControl=Selection of Reset will increase slice count due to use of real FFs and instead of SRLs  en=off  latency=1  dbl_ovrd=off  reg_retiming=on  block_type=delay
  din5_1 : xbsIndex_r4/Delay  rst=off  infoeditControl=Selection of Reset will increase slice count due to use of real FFs and instead of SRLs  en=off  latency=1  dbl_ovrd=off  reg_retiming=on  block_type=delay
  din6_0 : xbsIndex_r4/Delay  rst=off  infoeditControl=Selection of Reset will increase slice count due to use of real FFs and instead of SRLs  en=off  latency=1  dbl_ovrd=off  reg_retiming=on  block_type=delay
  din6_1 : xbsIndex_r4/Delay  rst=off  infoeditControl=Selection of Reset will increase slice count due to use of real FFs and instead of SRLs  en=off  latency=1  dbl_ovrd=off  reg_retiming=on  block_type=delay
  din7_0 : xbsIndex_r4/Delay  rst=off  infoeditControl=Selection of Reset will increase slice count due to use of real FFs and instead of SRLs  en=off  latency=1  dbl_ovrd=off  reg_retiming=on  block_type=delay
  din7_1 : xbsIndex_r4/Delay  rst=off  infoeditControl=Selection of Reset will increase slice count due to use of real FFs and instead of SRLs  en=off  latency=1  dbl_ovrd=off  reg_retiming=on  block_type=delay
  din8_0 : xbsIndex_r4/Delay  rst=off  infoeditControl=Selection of Reset will increase slice count due to use of real FFs and instead of SRLs  en=off  latency=1  dbl_ovrd=off  reg_retiming=off  block_type=delay
  din8_1 : xbsIndex_r4/Delay  rst=off  infoeditControl=Selection of Reset will increase slice count due to use of real FFs and instead of SRLs  en=off  latency=1  dbl_ovrd=off  reg_retiming=off  block_type=delay
  out : Outport
  wires:
  in/1 -> din0_0/1
  din0_0/1 -> din1_0/1, din1_1/1
  din1_0/1 -> din2_0/1
  din1_1/1 -> din2_1/1
  din2_0/1 -> din3_0/1
  din2_1/1 -> din3_1/1
  din3_0/1 -> din4_0/1
  din3_1/1 -> din4_1/1
  din4_0/1 -> din5_0/1
  din4_1/1 -> din5_1/1
  din5_0/1 -> din6_0/1
  din5_1/1 -> din6_1/1
  din6_0/1 -> din7_0/1
  din6_1/1 -> din7_1/1
  din7_0/1 -> din8_0/1
  din7_1/1 -> din8_1/1
  din8_0/1 -> bussify/1(in1)
  din8_1/1 -> bussify/2(in2)
  bussify/1(bus_out) -> out/1

== system pfb_fir_generic_test_sim3/pfb_fir_generic/pfb_fir_coeff_gen/en_replicate/bussify ==
  in1 : Inport
  in2 : Inport  Port=2
  in3 : Inport  Port=3
  in4 : Inport  Port=4
  in5 : Inport  Port=5
  in6 : Inport  Port=6
  in7 : Inport  Port=7
  in8 : Inport  Port=8
  in9 : Inport  Port=9
  in10 : Inport  Port=10
  in11 : Inport  Port=11
  in12 : Inport  Port=12
  in13 : Inport  Port=13
  in14 : Inport  Port=14
  in15 : Inport  Port=15
  in16 : Inport  Port=16
  in17 : Inport  Port=17
  in18 : Inport  Port=18
  in19 : Inport  Port=19
  in20 : Inport  Port=20
  in21 : Inport  Port=21
  in22 : Inport  Port=22
  in23 : Inport  Port=23
  in24 : Inport  Port=24
  in25 : Inport  Port=25
  concatenate : xbsIndex_r4/Concat  num_inputs=25  dbl_ovrd=off  block_type=concat
  reinterpret{1..25} (25 alike) : xbsIndex_r4/Reinterpret  force_arith_type=on  arith_type=Unsigned  force_bin_pt=on  bin_pt=0  block_type=reinterpret
      reinterpret1 settings: infoedit="Changes signal type without altering the binary representation.   You can changed the signal between signed and unsigned, and relocate the binary point.<br><br>Hardware notes: In hardware this block costs nothing.<br><br>Example:  Suppose the input is 6 bits wide, signed, with 2 fractional bits, and the output is forced to unsigned with 0 fractional bits.  Then an input of -2.0 (1110.00 in binary 2's complement) becomes an output of 56 (111000 in binary)."
      reinterpret2 settings: infoedit="Changes signal type without altering the binary representation.   You can changed the signal between signed and unsigned, and relocate the binary point.<br><br>Hardware notes: In hardware this block costs nothing.<br><br>Example:  Suppose the input is 6 bits wide, signed, with 2 fractional bits, and the output is forced to unsigned with 0 fractional bits.  Then an input of -2.0 (1110.00 in binary 2's complement) becomes an output of 56 (111000 in binary)."
  bus_out : Outport
  wires:
  concatenate/1 -> bus_out/1
  in1/1 -> reinterpret1/1
  reinterpret1/1 -> concatenate/1
  in2/1 -> reinterpret2/1
  reinterpret2/1 -> concatenate/2
  in3/1 -> reinterpret3/1
  reinterpret3/1 -> concatenate/3
  in4/1 -> reinterpret4/1
  reinterpret4/1 -> concatenate/4
  in5/1 -> reinterpret5/1
  reinterpret5/1 -> concatenate/5
  in6/1 -> reinterpret6/1
  reinterpret6/1 -> concatenate/6
  in7/1 -> reinterpret7/1
  reinterpret7/1 -> concatenate/7
  in8/1 -> reinterpret8/1
  reinterpret8/1 -> concatenate/8
  in9/1 -> reinterpret9/1
  reinterpret9/1 -> concatenate/9
  in10/1 -> reinterpret10/1
  reinterpret10/1 -> concatenate/10
  in11/1 -> reinterpret11/1
  reinterpret11/1 -> concatenate/11
  in12/1 -> reinterpret12/1
  reinterpret12/1 -> concatenate/12
  in13/1 -> reinterpret13/1
  reinterpret13/1 -> concatenate/13
  in14/1 -> reinterpret14/1
  reinterpret14/1 -> concatenate/14
  in15/1 -> reinterpret15/1
  reinterpret15/1 -> concatenate/15
  in16/1 -> reinterpret16/1
  reinterpret16/1 -> concatenate/16
  in17/1 -> reinterpret17/1
  reinterpret17/1 -> concatenate/17
  in18/1 -> reinterpret18/1
  reinterpret18/1 -> concatenate/18
  in19/1 -> reinterpret19/1
  reinterpret19/1 -> concatenate/19
  in20/1 -> reinterpret20/1
  reinterpret20/1 -> concatenate/20
  in21/1 -> reinterpret21/1
  reinterpret21/1 -> concatenate/21
  in22/1 -> reinterpret22/1
  reinterpret22/1 -> concatenate/22
  in23/1 -> reinterpret23/1
  reinterpret23/1 -> concatenate/23
  in24/1 -> reinterpret24/1
  reinterpret24/1 -> concatenate/24
  in25/1 -> reinterpret25/1
  reinterpret25/1 -> concatenate/25

== system pfb_fir_generic_test_sim3/pfb_fir_generic/pfb_fir_coeff_gen/munge/join ==
  in1 : Inport
  in2 : Inport  Port=2
  in3 : Inport  Port=3
  in4 : Inport  Port=4
  in5 : Inport  Port=5
  in6 : Inport  Port=6
  in7 : Inport  Port=7
  in8 : Inport  Port=8
  in9 : Inport  Port=9
  in10 : Inport  Port=10
  in11 : Inport  Port=11
  in12 : Inport  Port=12
  in13 : Inport  Port=13
  in14 : Inport  Port=14
  in15 : Inport  Port=15
  in16 : Inport  Port=16
  concatenate : xbsIndex_r4/Concat  num_inputs=16  dbl_ovrd=off  block_type=concat
  reinterpret{1..16} (16 alike) : xbsIndex_r4/Reinterpret  force_arith_type=on  arith_type=Unsigned  force_bin_pt=on  bin_pt=0  block_type=reinterpret
      reinterpret1 settings: infoedit="Changes signal type without altering the binary representation.   You can changed the signal between signed and unsigned, and relocate the binary point.<br><br>Hardware notes: In hardware this block costs nothing.<br><br>Example:  Suppose the input is 6 bits wide, signed, with 2 fractional bits, and the output is forced to unsigned with 0 fractional bits.  Then an input of -2.0 (1110.00 in binary 2's complement) becomes an output of 56 (111000 in binary)."
      reinterpret2 settings: infoedit="Changes signal type without altering the binary representation.   You can changed the signal between signed and unsigned, and relocate the binary point.<br><br>Hardware notes: In hardware this block costs nothing.<br><br>Example:  Suppose the input is 6 bits wide, signed, with 2 fractional bits, and the output is forced to unsigned with 0 fractional bits.  Then an input of -2.0 (1110.00 in binary 2's complement) becomes an output of 56 (111000 in binary)."
  bus_out : Outport
  wires:
  concatenate/1 -> bus_out/1
  in1/1 -> reinterpret1/1
  reinterpret1/1 -> concatenate/1
  in2/1 -> reinterpret2/1
  reinterpret2/1 -> concatenate/2
  in3/1 -> reinterpret3/1
  reinterpret3/1 -> concatenate/3
  in4/1 -> reinterpret4/1
  reinterpret4/1 -> concatenate/4
  in5/1 -> reinterpret5/1
  reinterpret5/1 -> concatenate/5
  in6/1 -> reinterpret6/1
  reinterpret6/1 -> concatenate/6
  in7/1 -> reinterpret7/1
  reinterpret7/1 -> concatenate/7
  in8/1 -> reinterpret8/1
  reinterpret8/1 -> concatenate/8
  in9/1 -> reinterpret9/1
  reinterpret9/1 -> concatenate/9
  in10/1 -> reinterpret10/1
  reinterpret10/1 -> concatenate/10
  in11/1 -> reinterpret11/1
  reinterpret11/1 -> concatenate/11
  in12/1 -> reinterpret12/1
  reinterpret12/1 -> concatenate/12
  in13/1 -> reinterpret13/1
  reinterpret13/1 -> concatenate/13
  in14/1 -> reinterpret14/1
  reinterpret14/1 -> concatenate/14
  in15/1 -> reinterpret15/1
  reinterpret15/1 -> concatenate/15
  in16/1 -> reinterpret16/1
  reinterpret16/1 -> concatenate/16

== system pfb_fir_generic_test_sim3/pfb_fir_generic/pfb_fir_coeff_gen/munge/split ==
  bus_in : Inport
  reinterpret{1..16} (16 alike) : xbsIndex_r4/Reinterpret  force_arith_type=on  arith_type=Unsigned  force_bin_pt=on  bin_pt=0  block_type=reinterpret
  slice1 : xbsIndex_r4/Slice  nbits=18  boolean_output=off  mode=Upper Bit Location + Width  bit1=-270  base1=MSB of Input  bit0=0  base0=LSB of Input  dbl_ovrd=off  block_type=slice
  slice10 : xbsIndex_r4/Slice  nbits=18  boolean_output=off  mode=Upper Bit Location + Width  bit1=-108  base1=MSB of Input  bit0=0  base0=LSB of Input  dbl_ovrd=off  block_type=slice
  slice11 : xbsIndex_r4/Slice  nbits=18  boolean_output=off  mode=Upper Bit Location + Width  bit1=-90  base1=MSB of Input  bit0=0  base0=LSB of Input  dbl_ovrd=off  block_type=slice
  slice12 : xbsIndex_r4/Slice  nbits=18  boolean_output=off  mode=Upper Bit Location + Width  bit1=-72  base1=MSB of Input  bit0=0  base0=LSB of Input  dbl_ovrd=off  block_type=slice
  slice13 : xbsIndex_r4/Slice  nbits=18  boolean_output=off  mode=Upper Bit Location + Width  bit1=-54  base1=MSB of Input  bit0=0  base0=LSB of Input  dbl_ovrd=off  block_type=slice
  slice14 : xbsIndex_r4/Slice  nbits=18  boolean_output=off  mode=Upper Bit Location + Width  bit1=-36  base1=MSB of Input  bit0=0  base0=LSB of Input  dbl_ovrd=off  block_type=slice
  slice15 : xbsIndex_r4/Slice  nbits=18  boolean_output=off  mode=Upper Bit Location + Width  bit1=-18  base1=MSB of Input  bit0=0  base0=LSB of Input  dbl_ovrd=off  block_type=slice
  slice16 : xbsIndex_r4/Slice  nbits=18  boolean_output=off  mode=Upper Bit Location + Width  bit1=0  base1=MSB of Input  bit0=0  base0=LSB of Input  dbl_ovrd=off  block_type=slice
  slice2 : xbsIndex_r4/Slice  nbits=18  boolean_output=off  mode=Upper Bit Location + Width  bit1=-252  base1=MSB of Input  bit0=0  base0=LSB of Input  dbl_ovrd=off  block_type=slice
  slice3 : xbsIndex_r4/Slice  nbits=18  boolean_output=off  mode=Upper Bit Location + Width  bit1=-234  base1=MSB of Input  bit0=0  base0=LSB of Input  dbl_ovrd=off  block_type=slice
  slice4 : xbsIndex_r4/Slice  nbits=18  boolean_output=off  mode=Upper Bit Location + Width  bit1=-216  base1=MSB of Input  bit0=0  base0=LSB of Input  dbl_ovrd=off  block_type=slice
  slice5 : xbsIndex_r4/Slice  nbits=18  boolean_output=off  mode=Upper Bit Location + Width  bit1=-198  base1=MSB of Input  bit0=0  base0=LSB of Input  dbl_ovrd=off  block_type=slice
  slice6 : xbsIndex_r4/Slice  nbits=18  boolean_output=off  mode=Upper Bit Location + Width  bit1=-180  base1=MSB of Input  bit0=0  base0=LSB of Input  dbl_ovrd=off  block_type=slice
  slice7 : xbsIndex_r4/Slice  nbits=18  boolean_output=off  mode=Upper Bit Location + Width  bit1=-162  base1=MSB of Input  bit0=0  base0=LSB of Input  dbl_ovrd=off  block_type=slice
  slice8 : xbsIndex_r4/Slice  nbits=18  boolean_output=off  mode=Upper Bit Location + Width  bit1=-144  base1=MSB of Input  bit0=0  base0=LSB of Input  dbl_ovrd=off  block_type=slice
  slice9 : xbsIndex_r4/Slice  nbits=18  boolean_output=off  mode=Upper Bit Location + Width  bit1=-126  base1=MSB of Input  bit0=0  base0=LSB of Input  dbl_ovrd=off  block_type=slice
  msb_out16 : Outport
  out15 : Outport  Port=2
  out14 : Outport  Port=3
  out13 : Outport  Port=4
  out12 : Outport  Port=5
  out11 : Outport  Port=6
  out10 : Outport  Port=7
  out9 : Outport  Port=8
  out8 : Outport  Port=9
  out7 : Outport  Port=10
  out6 : Outport  Port=11
  out5 : Outport  Port=12
  out4 : Outport  Port=13
  out3 : Outport  Port=14
  out2 : Outport  Port=15
  lsb_out1 : Outport  Port=16
  wires:
  bus_in/1 -> slice16/1, slice15/1, slice14/1, slice13/1, slice12/1, slice11/1, slice10/1, slice9/1, slice8/1, slice7/1, slice6/1, slice5/1, slice4/1, slice3/1, slice2/1, slice1/1
  slice16/1 -> reinterpret16/1
  reinterpret16/1 -> msb_out16/1
  slice15/1 -> reinterpret15/1
  reinterpret15/1 -> out15/1
  slice14/1 -> reinterpret14/1
  reinterpret14/1 -> out14/1
  slice13/1 -> reinterpret13/1
  reinterpret13/1 -> out13/1
  slice12/1 -> reinterpret12/1
  reinterpret12/1 -> out12/1
  slice11/1 -> reinterpret11/1
  reinterpret11/1 -> out11/1
  slice10/1 -> reinterpret10/1
  reinterpret10/1 -> out10/1
  slice9/1 -> reinterpret9/1
  reinterpret9/1 -> out9/1
  slice8/1 -> reinterpret8/1
  reinterpret8/1 -> out8/1
  slice7/1 -> reinterpret7/1
  reinterpret7/1 -> out7/1
  slice6/1 -> reinterpret6/1
  reinterpret6/1 -> out6/1
  slice5/1 -> reinterpret5/1
  reinterpret5/1 -> out5/1
  slice4/1 -> reinterpret4/1
  reinterpret4/1 -> out4/1
  slice3/1 -> reinterpret3/1
  reinterpret3/1 -> out3/1
  slice2/1 -> reinterpret2/1
  reinterpret2/1 -> out2/1
  slice1/1 -> reinterpret1/1
  reinterpret1/1 -> lsb_out1/1
